simulink model "Linear_Moving_Setpoint_SS"  (R2021a)
settings: Solver=VariableStepAuto  StartTime=tspan(1)  StopTime=tspan(2)  RelTol=1e-9
undefined symbols (not defined in the file): Aa, Ba, C, D, K, r_sim, S, x_s_select, xa_0
libraries: simulink_extras x1
settings Model: Creator=domin  LastModifiedBy=domin
settings SolverCC: AlgebraicLoopSolver=TrustRegion
settings DebuggingCC: SFMachineParentedDataDiag=warning

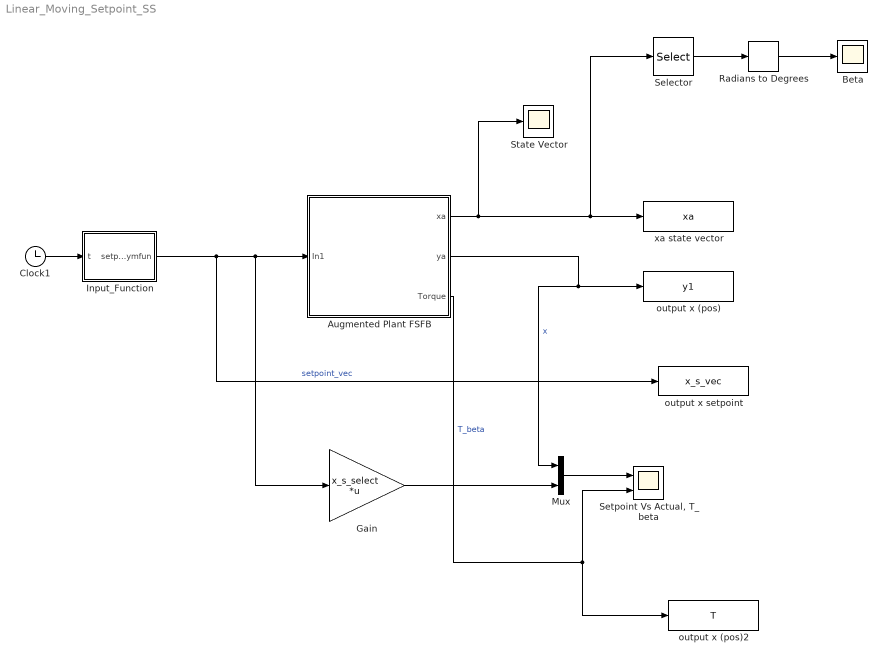
== system Linear_Moving_Setpoint_SS ==
  Augmented Plant FSFB : Subsystem
  Beta : Scope
  Clock1 : Clock
  Gain : Gain  Gain=x_s_select  Multiplication=Matrix(K*u)
  Input_Function : MATLAB Function  TreatAsAtomicUnit=on
  Mux : Mux  Inputs=2
  Radians to Degrees : simulink_extras/Transformations/Radians to Degrees
  Selector : Selector  InputPortWidth=5  IndexOptions=Index vector (dialog)  Indices=[2]  OutputSizes=1
  "Setpoint Vs Actual, T_beta" : Scope  NumInputPorts=2
  State Vector : Scope
  output x (pos) : ToWorkspace  VariableName=y1  SampleTime=-1
  output x (pos)2 : ToWorkspace  VariableName=T  SampleTime=-1
  output x setpoint : ToWorkspace  VariableName=x_s_vec  SampleTime=-1
  xa state vector : ToWorkspace  VariableName=xa  SampleTime=-1
  wires:
  Input_Function/1(setpoint_symfun) -> output x setpoint/1, Augmented Plant FSFB/1(In1), Gain/1  "setpoint_vec"
  Augmented Plant FSFB/2(ya) -> Mux/1, output x (pos)/1  "x"
  Augmented Plant FSFB/1(xa) -> Selector/1, xa state vector/1, State Vector/1
  Selector/1 -> Radians to Degrees/1
  Radians to Degrees/1 -> Beta/1
  Mux/1 -> "Setpoint Vs Actual, T_beta"/1
  Augmented Plant FSFB/3(Torque) -> output x (pos)2/1, "Setpoint Vs Actual, T_beta"/2  "T_beta"
  Gain/1 -> Mux/2
  Clock1/1 -> Input_Function/1(t)

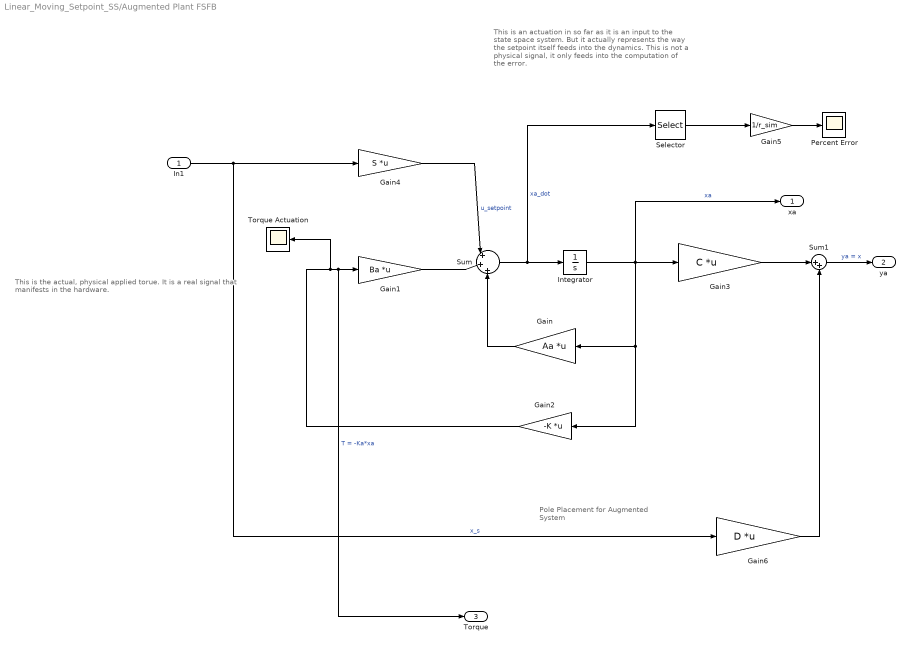
== system Linear_Moving_Setpoint_SS/Augmented Plant FSFB ==
  note: This is the actual, physical applied torue. It is a real signal
      | that manifests in the hardware.
  note: This is an actuation in so far as it is an input to the
      | state space system. But it actually represents the
      | way the setpoint itself feeds into the dynamics. This
      | is not a physical signal, it only feeds into the
      | computation of the error.
  note: Pole Placement for
      | Augmented System
  In1 : Inport
  Gain : Gain  Gain=Aa  Multiplication=Matrix(K*u)
  Gain1 : Gain  Gain=Ba  Multiplication=Matrix(K*u)
  Gain2 : Gain  Gain=-K  Multiplication=Matrix(K*u)
  Gain3 : Gain  Gain=C  Multiplication=Matrix(K*u)
  Gain4 : Gain  Gain=S  Multiplication=Matrix(K*u)
  Gain5 : Gain  Gain=1/r_sim
  Gain6 : Gain  Gain=D  Multiplication=Matrix(K*u)
  Integrator : Integrator  InitialCondition=xa_0
  Percent Error : Scope
  Selector : Selector  InputPortWidth=5  IndexOptions=Index vector (dialog)  Indices=[1]  OutputSizes=1
  Sum : Sum  Inputs=|+|+|+
  Sum1 : Sum  Inputs=|++
  Torque Actuation : Scope
  xa : Outport
  ya : Outport  Port=2
  Torque : Outport  Port=3
  wires:
  Gain1/1 -> Sum/2
  Sum/1 -> Selector/1, Integrator/1  "xa_dot"
  Integrator/1 -> xa/1, Gain2/1, Gain/1, Gain3/1  "xa"
  Gain3/1 -> Sum1/1
  Gain/1 -> Sum/3
  Gain2/1 -> Torque Actuation/1, Torque/1, Gain1/1  "T = -Ka*xa"
  In1/1 -> Gain4/1, Gain6/1  "x_s"
  Gain4/1 -> Sum/1  "u_setpoint"
  Gain5/1 -> Percent Error/1
  Selector/1 -> Gain5/1
  Sum1/1 -> ya/1  "ya = x"
  Gain6/1 -> Sum1/2

== matlab function Linear_Moving_Setpoint_SS/Input_Function ==
  data: t input; setpoint_symfun output
function setpoint_symfun = Input_Function(t)
%#codegen

%    This function was generated by the Symbolic Math Toolbox version 8.7.
%    27-Sep-2021 23:14:27

setpoint_symfun = sin((t.*pi)./2.0).*(exp(t.*(-5.0./4.0))-1.0).*-5.0e+1;
